simulink model "sampleModel1744_3_sub"  (R2023a)
settings: Solver=VariableStepAuto  StartTime=0.0  StopTime=10.0  RelTol=1e-3
libraries: hdlsllib x4, simulink x1
settings Model: Creator=user1  LastModifiedBy=user1

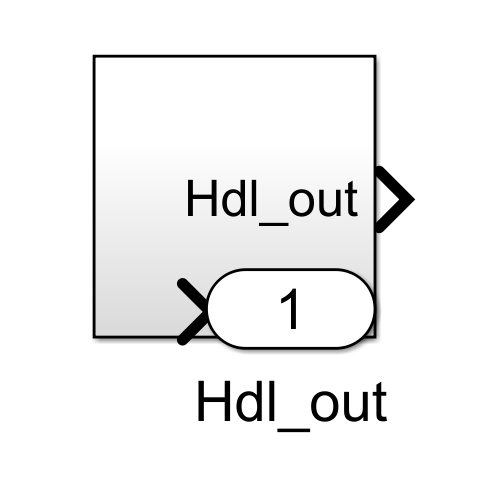
[thumbnail: Simulink's stored preview of the top-level diagram]
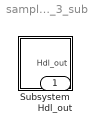
== system sampleModel1744_3_sub ==
  Subsystem : Subsystem
  Hdl_out : Outport  OutDataTypeStr=uint8

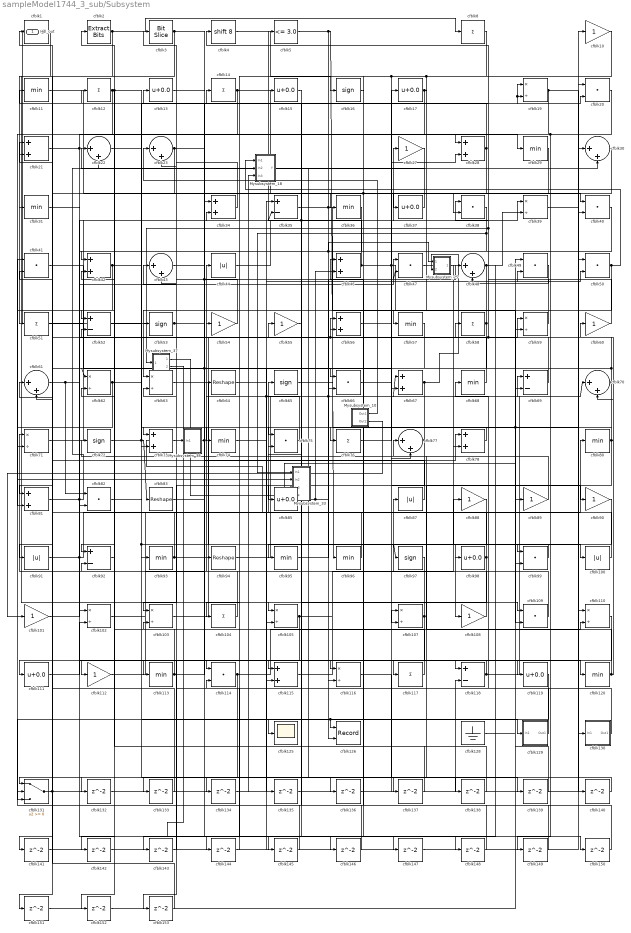
== system sampleModel1744_3_sub/Subsystem ==
  Mysubsystem_10 : Subsystem  TreatAsAtomicUnit=on  RTWFcnName=Mysubsystem_10
      settings: RTWFcnNameOpts=User specified  RTWFileNameOpts=Use function name
  Mysubsystem_18 : Subsystem  TreatAsAtomicUnit=on  RTWFcnName=Mysubsystem_18
      settings: RTWFcnNameOpts=User specified  RTWFileNameOpts=Use function name
  Mysubsystem_25 : Subsystem  TreatAsAtomicUnit=on  RTWFcnName=Mysubsystem_25
      settings: RTWFcnNameOpts=User specified  RTWFileNameOpts=Use function name
  Mysubsystem_33 : Subsystem  TreatAsAtomicUnit=on  RTWFcnName=Mysubsystem_33
      settings: RTWFcnNameOpts=User specified  RTWFileNameOpts=Use function name
  Mysubsystem_37 : Subsystem  TreatAsAtomicUnit=on  RTWFcnName=Mysubsystem_37
      settings: RTWFcnNameOpts=User specified  RTWFileNameOpts=Use function name
  Mysubsystem_38 : Subsystem  TreatAsAtomicUnit=on  RTWFcnName=Mysubsystem_38
      settings: RTWFcnNameOpts=User specified  RTWFileNameOpts=Use function name
  cfblk1 : hdlsllib/Logic and Bit Operations/Compare To Zero  relop=<=  OutDataTypeStr=uint8
  cfblk{10,27,54..55,60,88..90,101,108,112} (11 alike) : Gain  OutDataTypeStr=uint8
  cfblk{44,87,91,100} (4 alike) : Abs  OutDataTypeStr=uint8  SaturateOnIntegerOverflow=off
  cfblk{19,39,59,62..63,71,102..103,105,107,110,116} (12 alike) : Product  Inputs=*/  OutDataTypeStr=uint8  RndMeth=Zero  SaturateOnIntegerOverflow=on
  cfblk{8,12,14,51,58,76,104,117} (8 alike) : Sum  Inputs=+  OutDataTypeStr=uint8
  cfblk{20,38,40..41,47,49..50,66,75,82,99,109,114} (13 alike) : DotProduct  OutDataTypeStr=uint8
  cfblk{11,29,31,36,57,68,74,80,93,95..96,113,120} (13 alike) : MinMax  OutDataTypeStr=uint8
  cfblk{13,15,17,37,85,98,111,119} (8 alike) : Bias  Bias=0.0  SaturateOnIntegerOverflow=off
  cfblk{21,28,34,42,46,56,67,73,78,81,115} (11 alike) : Sum  OutDataTypeStr=uint8
  cfblk{35,52,69,92,118} (5 alike) : Sum  Inputs=+-  OutDataTypeStr=uint8
  cfblk125 : Scope
  cfblk126 : Record  FileSettingsInternal="{\"entries\":[{\"content\":{\"excelSettings\":{\"content\":{},\"type\":\"Streamout.ExcelSettings\"}},\"type\":\"Streamout.FileSettingStorage\",\"uuid\":\"\"}],\"packageUris\":[\"http:\\/\\/schema.mathworks.com\\/mf0\\/streamout_blocks\\/R2020a\"],\"version\":\"1.0\"}"  Layout=[1 1]  SignalsInternal="{\"entries\":[{\"content\":{\"signals\":[{\"content\":{\"blockPath\":[],\"dimensions\":[1],\"domain\":\"\",\"lineColor\":\"#a2142f\",\"plots\":[1],\"port\":1,\"signalID\":38904,\"signalName\":\"cfblk119\"},\"type\":\"RecordBlkView.Signal\",\"uuid\":\"\"},{\"content\":{\"blockPath\":[],\"dimensions\":[1],\"domain\":\"\",\"lineColor\":\"#139fff\",\"plots\":[1],\"port\":2,\"signalID\":38907,\"signalName\":\"cfblk19\"},\"type\":\"RecordBlkView.Signal\",\"uuid\":\"\"}]},\"type\":\"RecordBlkView.InputSignals\",\"uuid\":\"\"}],\"packageUris\":[\"http:\\/\\/schema.mathworks.com\\/mf0\\/streamout_blocks\\/R2020a\"],\"version\":\"1.0\"}"  VisualizationBindings="{\"xyplotplugin\":{\"info\":[{\"series\":[{\"bindingParametersList\":[{\"parameter\":\"X-Axis\",\"signalID\":38904,\"signalName\":\"cfblk119\"},{\"parameter\":\"Y-Axis\",\"signalID\":38907,\"signalName\":\"cfblk19\"}],\"seriesID\":43738}],\"subplotID\":1}]}}"  CompatibilityTag=XY  st=-1
  cfblk128 : Ground
  cfblk129 : Subsystem
      settings: LibrarySourceBlock=|
      | hdlsllib/Ports &
      | Subsystems/Subsystem
  cfblk130 : Subsystem
      settings: LibrarySourceBlock=|
      | hdlsllib/Ports &
      | Subsystems/Subsystem
  cfblk131 : Switch  OutDataTypeStr=uint8  SaturateOnIntegerOverflow=off  InputSameDT=off
  cfblk{132..153} (22 alike) : Delay  SampleTime=1
  cfblk{16,53,65,72,97} (5 alike) : Signum
  cfblk2 : simulink/Logic and Bit Operations/Extract Bits  bitsToExtract=Upper half  numBits=8  bitIdxRange=[0 7]  outScalingMode=Preserve fixed-point scaling
      settings: LibrarySourceBlock=|
      | hdlsllib/Logic and Bit
      | Operations/Extract Bits
  cfblk{22..23,30,43,48,61,70,77} (8 alike) : Sum  Inputs=|++  OutDataTypeStr=uint8
  cfblk3 : hdlsllib/Logic and Bit Operations/Bit Slice  lidx=7  ridx=0
  cfblk4 : ArithShift  BitShiftNumber=8
  cfblk5 : hdlsllib/Logic and Bit Operations/Compare To Constant  relop=<=  const=3.0  OutDataTypeStr=uint8
  cfblk64 : Reshape
  cfblk83 : Reshape
  cfblk94 : Reshape
  Hdl_out : Outport  OutDataTypeStr=uint8
  wires:
  cfblk91/1 -> cfblk34/2, cfblk80/1
  cfblk90/1 -> cfblk108/1
  cfblk1/1 -> cfblk105/1
  cfblk68/1 -> cfblk43/2
  cfblk34/1 -> cfblk13/1
  cfblk110/1 -> cfblk112/1
  cfblk71/1 -> cfblk27/1
  cfblk5/1 -> cfblk28/1, cfblk96/1
  cfblk63/1 -> cfblk98/1
  cfblk89/1 -> cfblk72/1
  cfblk48/1 -> cfblk39/2, cfblk63/1
  cfblk93/1 -> cfblk21/2, cfblk55/1
  cfblk69/1 -> cfblk21/1, cfblk56/1
  cfblk85/1 -> cfblk46/2, cfblk67/1, cfblk48/1
  cfblk58/1 -> cfblk115/2, cfblk53/1
  cfblk31/1 -> cfblk102/1
  cfblk100/1 -> cfblk44/1
  cfblk36/1 -> cfblk42/1
  cfblk70/1 -> cfblk62/1, cfblk46/1, cfblk38/1, cfblk78/2, Mysubsystem_33/3(In3)
  cfblk77/1 -> cfblk103/1, cfblk76/1
  cfblk119/1 -> cfblk131/3, cfblk126/1
  cfblk40/1 -> cfblk82/2, Mysubsystem_25/1(In1)
  cfblk65/1 -> cfblk130/1(In1)
  cfblk14/1 -> cfblk38/2, cfblk51/1
  cfblk4/1 -> cfblk16/1
  cfblk11/1 -> cfblk40/1
  cfblk98/1 -> cfblk125/1, cfblk62/2
  cfblk46/1 -> cfblk5/1, cfblk28/2, cfblk109/2
  cfblk115/1 -> cfblk87/1
  cfblk2/1 -> cfblk141/1, cfblk8/1
  cfblk72/1 -> cfblk20/2, cfblk83/1
  cfblk95/1 -> cfblk69/1
  cfblk118/1 -> cfblk111/1, cfblk10/1
  cfblk75/1 -> cfblk54/1
  cfblk112/1 -> cfblk65/1
  cfblk129/1(Out1) -> cfblk23/2
  cfblk37/1 -> cfblk22/1
  cfblk44/1 -> cfblk39/1
  cfblk131/1 -> cfblk41/2, Mysubsystem_18/3(In3)
  cfblk120/1 -> cfblk70/2, cfblk77/1
  cfblk104/1 -> cfblk71/1
  cfblk52/1 -> cfblk97/1, cfblk118/1
  cfblk94/1 -> cfblk20/1
  cfblk80/1 -> cfblk137/1, cfblk60/1, cfblk73/1
  cfblk76/1 -> cfblk49/2
  cfblk103/1 -> cfblk59/1
  cfblk53/1 -> Hdl_out/1, cfblk120/1
  cfblk47/1 -> cfblk100/1
  cfblk61/1 -> cfblk82/1, cfblk114/1
  cfblk101/1 -> cfblk58/1
  cfblk114/1 -> cfblk153/1, cfblk110/2
  cfblk41/1 -> cfblk77/2
  cfblk109/1 -> cfblk64/1
  cfblk30/1 -> cfblk52/1
  cfblk3/1 -> cfblk148/1, cfblk31/1
  cfblk113/1 -> cfblk52/2, cfblk78/1
  cfblk88/1 -> cfblk115/1
  cfblk67/1 -> cfblk73/2, Mysubsystem_25/2(In2)
  cfblk29/1 -> cfblk146/1, cfblk92/1
  cfblk60/1 -> cfblk4/1
  cfblk57/1 -> cfblk91/1
  cfblk51/1 -> cfblk93/1
  cfblk17/1 -> cfblk81/2, cfblk57/1
  cfblk99/1 -> cfblk95/1
  cfblk35/1 -> cfblk117/1, cfblk89/1
  cfblk16/1 -> cfblk116/1
  cfblk20/1 -> cfblk149/1, cfblk74/1
  cfblk19/1 -> cfblk126/2, cfblk50/1
  cfblk38/1 -> cfblk144/1, Mysubsystem_33/1(In1)
  cfblk50/1 -> cfblk136/1, Mysubsystem_18/1(In1)
  cfblk54/1 -> cfblk3/1
  cfblk73/1 -> cfblk109/1, cfblk19/2, cfblk19/1
  cfblk62/1 -> cfblk30/2, Mysubsystem_33/2(In2)
  cfblk27/1 -> cfblk22/2
  cfblk117/1 -> cfblk12/1
  cfblk78/1 -> cfblk75/1
  cfblk97/1 -> cfblk92/2
  cfblk111/1 -> cfblk102/2
  cfblk15/1 -> cfblk85/1
  cfblk43/1 -> cfblk47/2, cfblk67/2, cfblk99/1
  cfblk59/1 -> Mysubsystem_37/1(In1), cfblk11/1
  cfblk108/1 -> cfblk15/1, cfblk35/2
  cfblk23/1 -> cfblk81/1, cfblk94/1
  cfblk21/1 -> cfblk147/1, cfblk29/1
  cfblk56/1 -> cfblk90/1
  cfblk66/1 -> cfblk17/1
  cfblk105/1 -> cfblk113/1, cfblk88/1
  cfblk74/1 -> cfblk70/1, cfblk50/2
  cfblk8/1 -> cfblk36/1
  cfblk128/1 -> cfblk59/2
  cfblk42/1 -> cfblk66/2, cfblk71/2
  cfblk83/1 -> cfblk119/1
  cfblk28/1 -> cfblk14/1, cfblk116/2
  cfblk10/1 -> cfblk37/1, cfblk104/1, cfblk107/2
  cfblk130/1(Out1) -> cfblk68/1
  cfblk82/1 -> cfblk129/1(In1)
  cfblk49/1 -> cfblk48/2
  cfblk12/1 -> cfblk151/1, cfblk152/1, cfblk66/1
  cfblk102/1 -> cfblk34/1
  cfblk81/1 -> cfblk47/1, Mysubsystem_18/2(In2)
  cfblk107/1 -> cfblk133/1, cfblk2/1
  cfblk87/1 -> cfblk61/1
  cfblk132/1 -> cfblk35/1
  cfblk133/1 -> cfblk1/1
  cfblk22/1 -> cfblk134/1
  cfblk134/1 -> cfblk107/1
  cfblk64/1 -> cfblk135/1
  cfblk135/1 -> cfblk118/2
  cfblk136/1 -> cfblk30/1
  cfblk137/1 -> cfblk42/2
  cfblk116/1 -> cfblk138/1
  cfblk138/1 -> cfblk63/2
  cfblk13/1 -> cfblk139/1
  cfblk139/1 -> cfblk49/1
  cfblk39/1 -> cfblk140/1
  cfblk140/1 -> cfblk131/1
  cfblk141/1 -> cfblk105/2
  cfblk92/1 -> cfblk142/1
  cfblk142/1 -> cfblk110/1
  cfblk143/1 -> cfblk43/1
  cfblk144/1 -> cfblk114/2
  cfblk55/1 -> cfblk145/1
  cfblk145/1 -> cfblk41/1
  cfblk146/1 -> cfblk131/2
  cfblk147/1 -> cfblk40/2
  cfblk148/1 -> cfblk75/2
  cfblk149/1 -> cfblk103/2
  cfblk150/1 -> cfblk56/2
  cfblk151/1 -> cfblk69/2
  cfblk152/1 -> cfblk99/2
  cfblk153/1 -> cfblk61/2
  Mysubsystem_10/1(Out1) -> cfblk23/1
  Mysubsystem_10/2(Out2) -> cfblk101/1
  Mysubsystem_18/1(Y) -> cfblk132/1
  Mysubsystem_25/1(Out1) -> cfblk143/1
  Mysubsystem_37/1(Out1) -> Mysubsystem_33/4(In4)
  Mysubsystem_37/2(Out2) -> cfblk150/1
  cfblk96/1 -> Mysubsystem_38/1(In1)

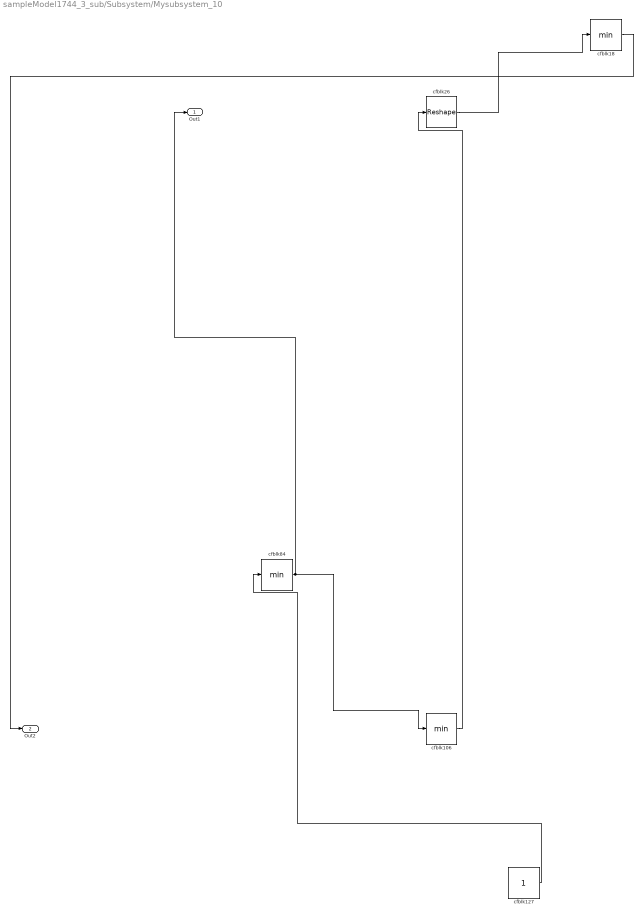
== system sampleModel1744_3_sub/Subsystem/Mysubsystem_10 ==
  cfblk106 : MinMax
  cfblk127 : Constant  SampleTime=-1
  cfblk18 : MinMax
  cfblk26 : Reshape
  cfblk84 : MinMax
  Out1 : Outport
  Out2 : Outport  Port=2
  wires:
  cfblk18/1 -> Out2/1
  cfblk26/1 -> cfblk18/1
  cfblk84/1 -> cfblk106/1, Out1/1
  cfblk127/1 -> cfblk84/1
  cfblk106/1 -> cfblk26/1

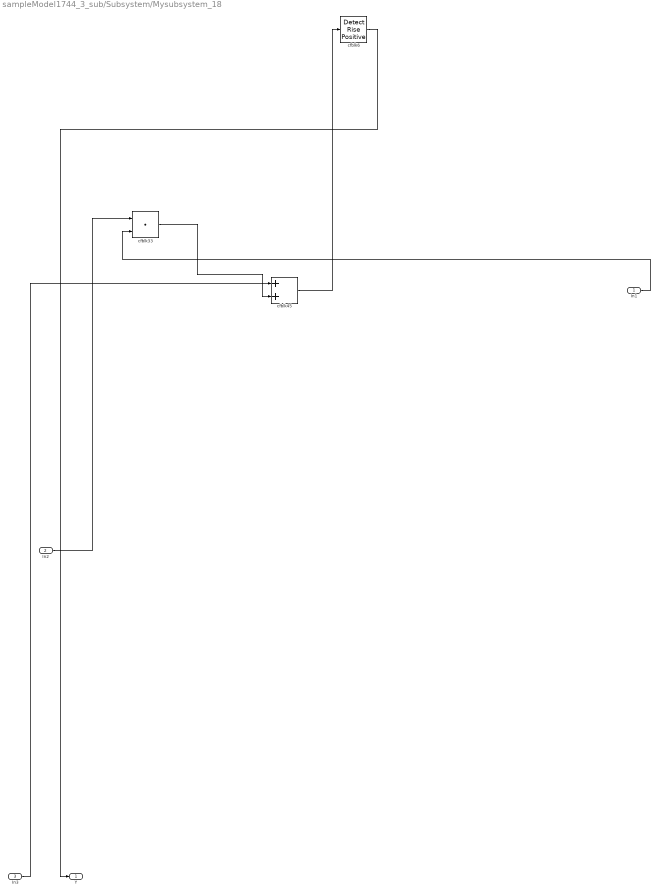
== system sampleModel1744_3_sub/Subsystem/Mysubsystem_18 ==
  In1 : Inport
  In2 : Inport  Port=2
  In3 : Inport  Port=3
  cfblk33 : DotProduct  OutDataTypeStr=Inherit: Inherit via internal rule
  cfblk45 : Sum
  cfblk6 : hdlsllib/Logic and Bit Operations/Detect Rise Positive  vinit=0  OutDataTypeStr=boolean
  Y : Outport
  wires:
  In1/1 -> cfblk33/2
  In3/1 -> cfblk45/1
  cfblk33/1 -> cfblk45/2
  cfblk45/1 -> cfblk6/1
  In2/1 -> cfblk33/1
  cfblk6/1 -> Y/1

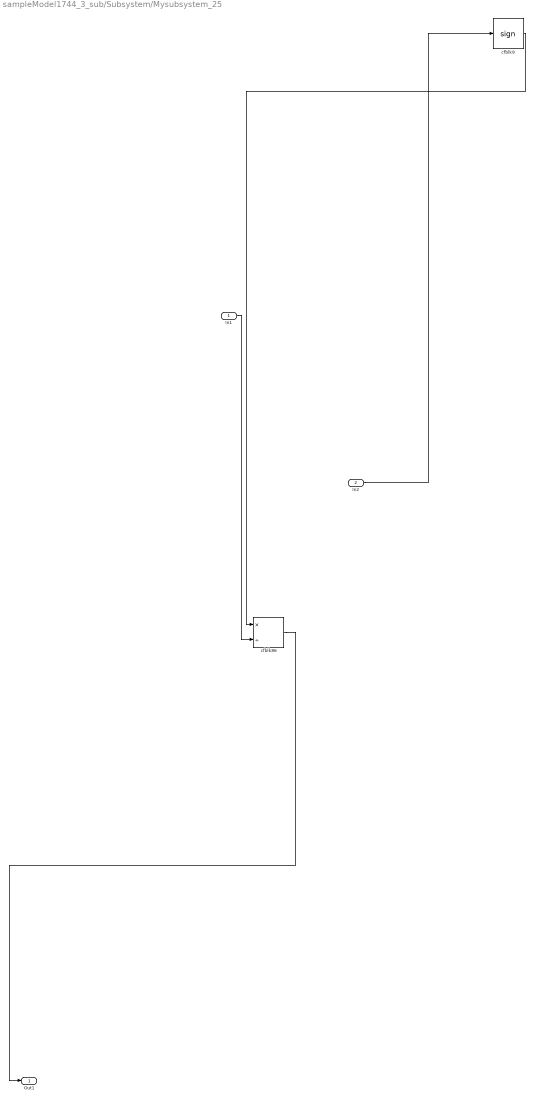
== system sampleModel1744_3_sub/Subsystem/Mysubsystem_25 ==
  In1 : Inport
  In2 : Inport  Port=2
  cfblk86 : Product  Inputs=*/  RndMeth=Zero  SaturateOnIntegerOverflow=on
  cfblk9 : Signum
  Out1 : Outport
  wires:
  In1/1 -> cfblk86/2
  cfblk86/1 -> Out1/1
  In2/1 -> cfblk9/1
  cfblk9/1 -> cfblk86/1

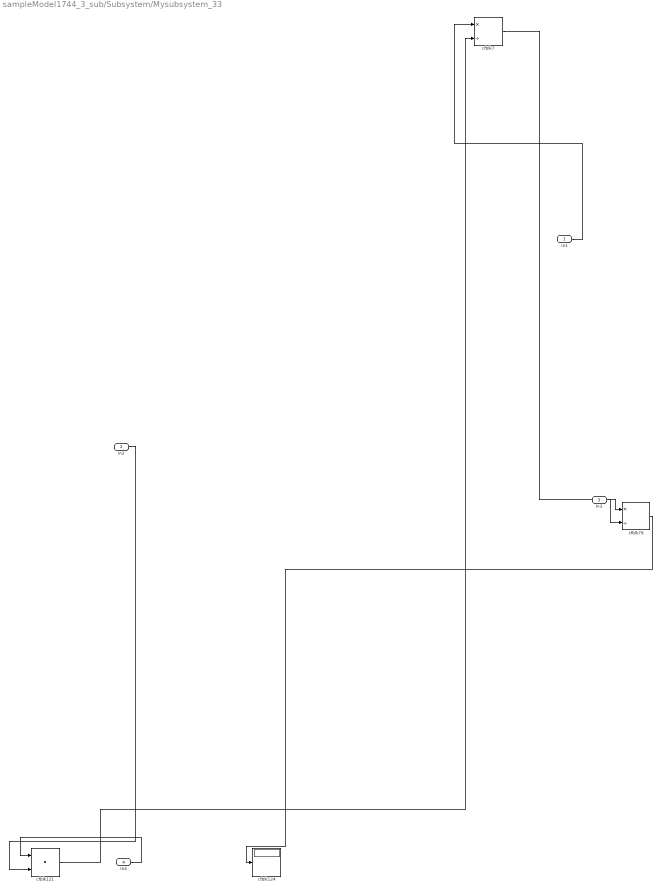
== system sampleModel1744_3_sub/Subsystem/Mysubsystem_33 ==
  In1 : Inport
  In2 : Inport  Port=2
  In3 : Inport  Port=3
  In4 : Inport  Port=4
  cfblk121 : DotProduct  OutDataTypeStr=Inherit: Inherit via internal rule
  cfblk124 : Display
  cfblk7 : Product  Inputs=*/  RndMeth=Zero  SaturateOnIntegerOverflow=on
  cfblk79 : Product  Inputs=*/  RndMeth=Zero  SaturateOnIntegerOverflow=on
  wires:
  In4/1 -> cfblk121/1
  In3/1 -> cfblk79/2
  In2/1 -> cfblk121/2
  In1/1 -> cfblk7/1
  cfblk7/1 -> cfblk79/1
  cfblk121/1 -> cfblk7/2
  cfblk79/1 -> cfblk124/1

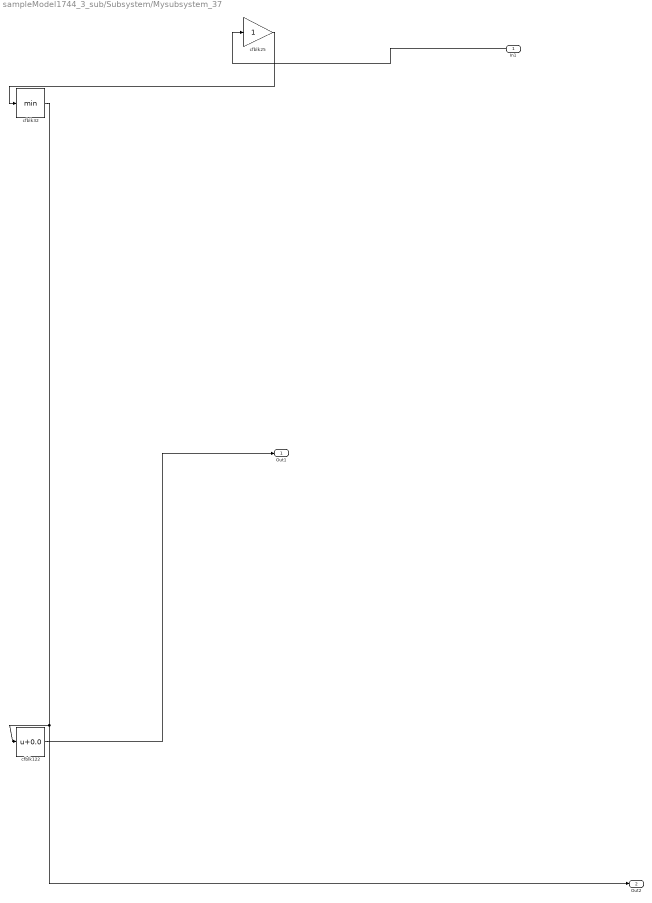
== system sampleModel1744_3_sub/Subsystem/Mysubsystem_37 ==
  In1 : Inport
  cfblk122 : Bias  Bias=0.0  SaturateOnIntegerOverflow=off
  cfblk25 : Gain
  cfblk32 : MinMax
  Out1 : Outport
  Out2 : Outport  Port=2
  wires:
  cfblk122/1 -> Out1/1
  In1/1 -> cfblk25/1
  cfblk25/1 -> cfblk32/1
  cfblk32/1 -> cfblk122/1, Out2/1

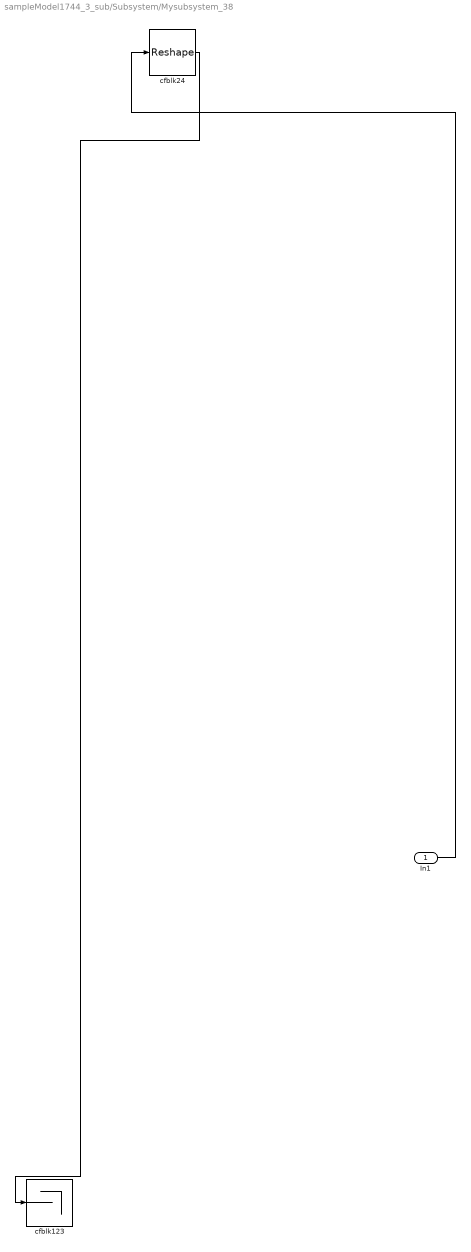
== system sampleModel1744_3_sub/Subsystem/Mysubsystem_38 ==
  In1 : Inport
  cfblk123 : Terminator
  cfblk24 : Reshape
  wires:
  In1/1 -> cfblk24/1
  cfblk24/1 -> cfblk123/1

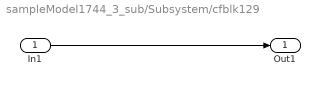
== system sampleModel1744_3_sub/Subsystem/cfblk129 ==
  In1 : Inport
  Out1 : Outport
  wires:
  In1/1 -> Out1/1

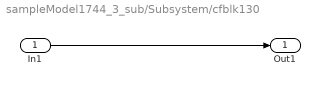
== system sampleModel1744_3_sub/Subsystem/cfblk130 ==
  In1 : Inport
  Out1 : Outport
  wires:
  In1/1 -> Out1/1
